simulink model "TV_LQR"  (R2024a)
settings: Solver=ode45  StartTime=0.0  StopTime=5*2.7499  MaxStep=0.001  RelTol=1e-10  AbsTol=1e-12
values from neighbouring files (symbols this model uses):
  K_all = zeros(3,6,N)    [time_varying_K_t.m]
  t_ref = data(:,1)    [compute_K.m]    (also in time_varying_K_t.m)
  t_vec = t_sol    [time_varying_K_t.m]
  vx_ref = X(:,4)    [compute_K.m]    (also in time_varying_K_t.m = X_ref(:,4))
  vy_ref = X(:,5)    [compute_K.m]    (also in time_varying_K_t.m = X_ref(:,5))
  vz_ref = X(:,6)    [compute_K.m]    (also in time_varying_K_t.m = X_ref(:,6))
  x0 = X(1,:)'    [compute_K.m]    (also in continuation.m = [r0;v0]; controlled_and_reference_orbit.m = [r0;v0]; halo_orbit_richardson.m = [r0;v0]; time_varying_K_t.m = X_ref(1,:)')
  x_ref = X(:,1)    [compute_K.m]    (also in time_varying_K_t.m = X_ref(:,1))
  y_ref = X(:,2)    [compute_K.m]    (also in time_varying_K_t.m = X_ref(:,2))
  z_ref = X(:,3)    [compute_K.m]    (also in time_varying_K_t.m = X_ref(:,3))
libraries: simulink x6
settings Model: Creator=MEGHNA  LastModifiedBy=MEGHNA
settings SolverCC: AutoScaleAbsTol=off

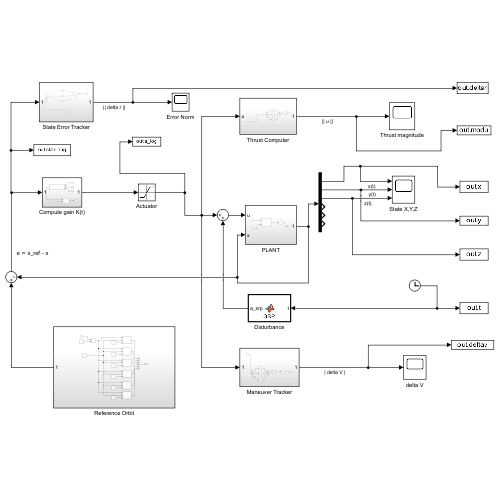
[thumbnail: Simulink's stored preview of the top-level diagram]
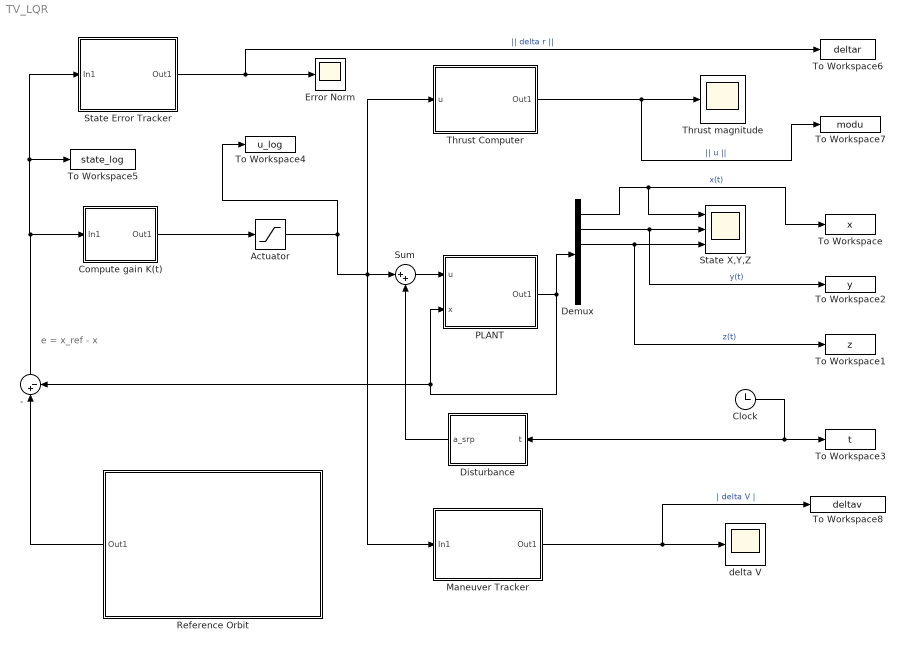
== system TV_LQR ==
  note: e = x_ref - x
  - : Sum  Inputs=|+-
  Actuator : Saturate  UpperLimit=5e-4  LowerLimit=-5e-4  LinearizeAsGain=off
  Clock : Clock
  Compute gain K(t) : Subsystem
  Demux : Demux  Outputs=6
  Disturbance : MATLAB Function  TreatAsAtomicUnit=on
  Error Norm : Scope
  Maneuver Tracker : Subsystem
  PLANT : Subsystem
  Reference Orbit : Subsystem
  State Error Tracker : Subsystem
  State X,Y,Z : Scope  NumInputPorts=3
  Sum : Sum  Inputs=|++
  Thrust Computer : Subsystem
  Thrust magnitude : Scope
  To Workspace : ToWorkspace  VariableName=x  SampleTime=-1
  To Workspace1 : ToWorkspace  VariableName=z  SampleTime=-1
  To Workspace2 : ToWorkspace  VariableName=y  SampleTime=-1
  To Workspace3 : ToWorkspace  VariableName=t  SampleTime=-1
  To Workspace4 : ToWorkspace  VariableName=u_log  SampleTime=-1
  To Workspace5 : ToWorkspace  VariableName=state_log  SampleTime=-1
  To Workspace6 : ToWorkspace  VariableName=deltar  SampleTime=-1
  To Workspace7 : ToWorkspace  VariableName=modu  SampleTime=-1
  To Workspace8 : ToWorkspace  VariableName=deltav  SampleTime=-1
  delta V : Scope
  wires:
  -/1 -> State Error Tracker/1(In1), To Workspace5/1, Compute gain K(t)/1(In1)
  Demux/1 -> To Workspace/1, State X,Y,Z/1  "x(t)"
  Demux/2 -> To Workspace2/1, State X,Y,Z/2  "y(t)"
  Demux/3 -> To Workspace1/1, State X,Y,Z/3  "z(t)"
  State Error Tracker/1(Out1) -> To Workspace6/1, Error Norm/1  "|| delta r ||"
  Maneuver Tracker/1(Out1) -> To Workspace8/1, delta V/1  "| delta V |"
  Actuator/1 -> Maneuver Tracker/1(In1), Sum/1, Thrust Computer/1(u), To Workspace4/1
  Thrust Computer/1(Out1) -> To Workspace7/1, Thrust magnitude/1  "|| u ||"
  Reference Orbit/1(Out1) -> -/1
  Clock/1 -> Disturbance/1(t), To Workspace3/1
  Sum/1 -> PLANT/1(u)
  Disturbance/1(a_srp) -> Sum/2
  PLANT/1(Out1) -> Demux/1, PLANT/2(x), -/2
  Compute gain K(t)/1(Out1) -> Actuator/1

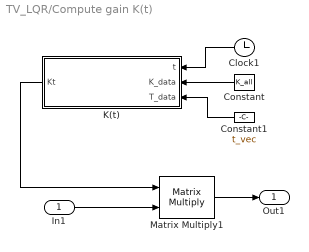
== system TV_LQR/Compute gain K(t) ==
  In1 : Inport
  Clock1 : Clock
  Constant : Constant  Value=K_all  SampleTime=-1
  Constant1 : Constant  Value=t_vec  SampleTime=-1
  K(t) : MATLAB Function  TreatAsAtomicUnit=on  SystemSampleTime=0.002
  Matrix Multiply1 : Product  Multiplication=Matrix(*)
  Out1 : Outport
  wires:
  Clock1/1 -> K(t)/1(t)
  In1/1 -> Matrix Multiply1/2
  Matrix Multiply1/1 -> Out1/1
  K(t)/1(Kt) -> Matrix Multiply1/1
  Constant/1 -> K(t)/2(K_data)
  Constant1/1 -> K(t)/3(T_data)

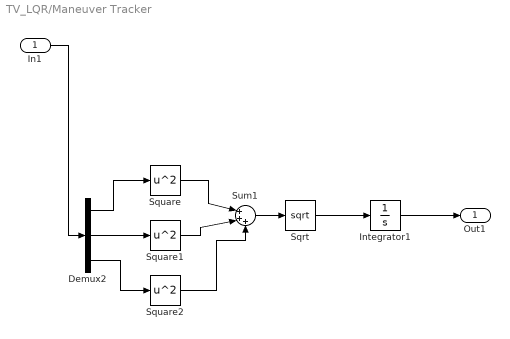
== system TV_LQR/Maneuver Tracker ==
  In1 : Inport
  Demux2 : Demux  Outputs=3
  Integrator1 : Integrator
  Sqrt : Sqrt
  Square : Math  Operator=square
  Square1 : Math  Operator=square
  Square2 : Math  Operator=square
  Sum1 : Sum  Inputs=|+++
  Out1 : Outport
  wires:
  Demux2/2 -> Square1/1
  Demux2/1 -> Square/1
  Square2/1 -> Sum1/3
  Square1/1 -> Sum1/2
  Sum1/1 -> Sqrt/1
  Square/1 -> Sum1/1
  Demux2/3 -> Square2/1
  Sqrt/1 -> Integrator1/1
  In1/1 -> Demux2/1
  Integrator1/1 -> Out1/1

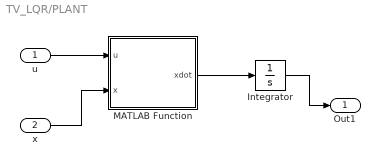
== system TV_LQR/PLANT ==
  u : Inport
  x : Inport  Port=2
  Integrator : Integrator  InitialCondition=x0
  MATLAB Function : MATLAB Function  TreatAsAtomicUnit=on
  Out1 : Outport
  wires:
  MATLAB Function/1(xdot) -> Integrator/1
  x/1 -> MATLAB Function/2(x)
  Integrator/1 -> Out1/1
  u/1 -> MATLAB Function/1(u)

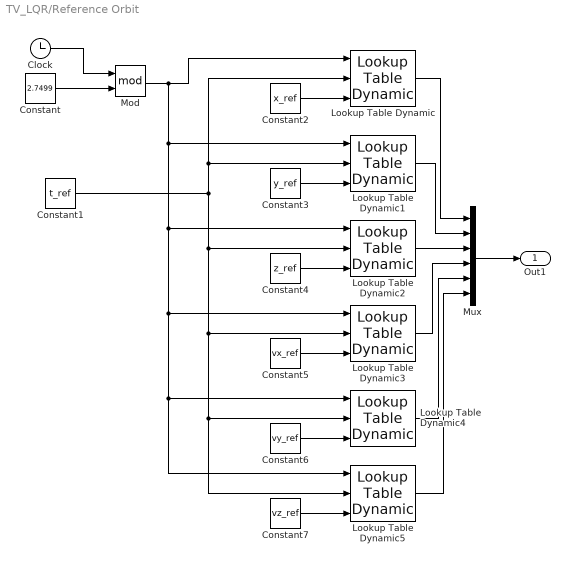
== system TV_LQR/Reference Orbit ==
  Clock : Clock
  Constant : Constant  Value=2.7499
  Constant1 : Constant  Value=t_ref
  Constant2 : Constant  Value=x_ref
  Constant3 : Constant  Value=y_ref
  Constant4 : Constant  Value=z_ref
  Constant5 : Constant  Value=vx_ref
  Constant6 : Constant  Value=vy_ref
  Constant7 : Constant  Value=vz_ref
  Lookup Table Dynamic{,1..5} (6 alike) : simulink/Lookup Tables/Lookup Table Dynamic  LookUpMeth=Interpolation-Use End Values  OutDataType=fixdt('double')  OutScaling=[]  OutputDataTypeScalingMode=Specify via dialog  OutDataTypeStr=double  DoSatur=off
  Mod : Math  Operator=mod
  Mux : Mux  Inputs=6
  Out1 : Outport
  wires:
  Lookup Table Dynamic4/1 -> Mux/5
  Constant5/1 -> Lookup Table Dynamic3/3
  Constant1/1 -> Lookup Table Dynamic5/2, Lookup Table Dynamic4/2, Lookup Table Dynamic3/2, Lookup Table Dynamic2/2, Lookup Table Dynamic1/2, Lookup Table Dynamic/2
  Lookup Table Dynamic1/1 -> Mux/2
  Mod/1 -> Lookup Table Dynamic5/1, Lookup Table Dynamic4/1, Lookup Table Dynamic3/1, Lookup Table Dynamic2/1, Lookup Table Dynamic1/1, Lookup Table Dynamic/1
  Lookup Table Dynamic/1 -> Mux/1
  Lookup Table Dynamic2/1 -> Mux/3
  Constant2/1 -> Lookup Table Dynamic/3
  Constant3/1 -> Lookup Table Dynamic1/3
  Constant4/1 -> Lookup Table Dynamic2/3
  Lookup Table Dynamic3/1 -> Mux/4
  Mux/1 -> Out1/1
  Constant6/1 -> Lookup Table Dynamic4/3
  Constant7/1 -> Lookup Table Dynamic5/3
  Lookup Table Dynamic5/1 -> Mux/6
  Clock/1 -> Mod/1
  Constant/1 -> Mod/2

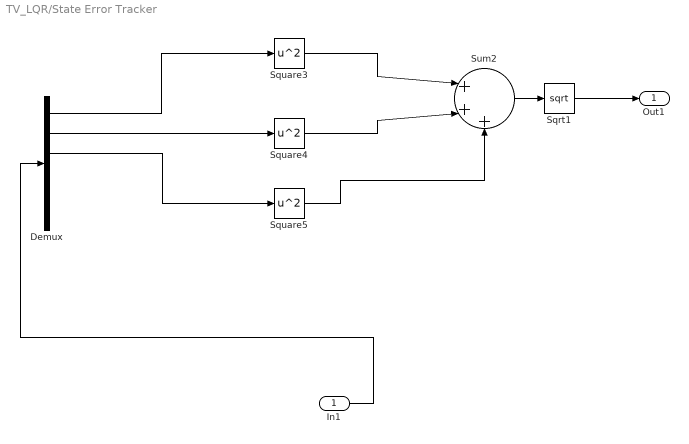
== system TV_LQR/State Error Tracker ==
  In1 : Inport
  Demux : Demux  Outputs=6
  Sqrt1 : Sqrt
  Square3 : Math  Operator=square
  Square4 : Math  Operator=square
  Square5 : Math  Operator=square
  Sum2 : Sum  Inputs=|+++
  Out1 : Outport
  wires:
  Square4/1 -> Sum2/2
  Sum2/1 -> Sqrt1/1
  Demux/2 -> Square4/1
  Demux/3 -> Square5/1
  Square3/1 -> Sum2/1
  Demux/1 -> Square3/1
  Square5/1 -> Sum2/3
  In1/1 -> Demux/1
  Sqrt1/1 -> Out1/1

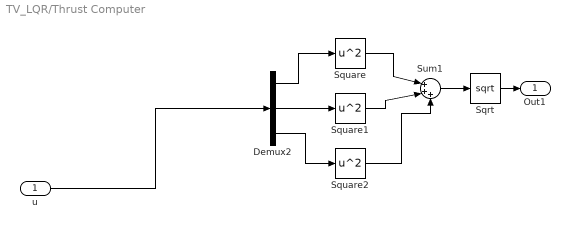
== system TV_LQR/Thrust Computer ==
  u : Inport
  Demux2 : Demux  Outputs=3
  Sqrt : Sqrt
  Square : Math  Operator=square
  Square1 : Math  Operator=square
  Square2 : Math  Operator=square
  Sum1 : Sum  Inputs=|+++
  Out1 : Outport
  wires:
  Square/1 -> Sum1/1
  u/1 -> Demux2/1
  Square2/1 -> Sum1/3
  Square1/1 -> Sum1/2
  Demux2/3 -> Square2/1
  Sum1/1 -> Sqrt/1
  Demux2/2 -> Square1/1
  Demux2/1 -> Square/1
  Sqrt/1 -> Out1/1

== matlab function TV_LQR/Compute gain K(t)/K(t) ==
  settings: updateMethod=DISCRETE  sampleTime=0.002
  data: t input size=1; Kt output size=[3 6]; K_data input size=[3 6 305]; T_data input size=[305 1]
function Kt = compute_K(t, K_data, T_data)
%#codegen

% --- FORCE FIXED OUTPUT SIZE ---
Kt = zeros(3,6);

N = 305;   % <-- HARD-CODE THIS (IMPORTANT)

T_final = T_data(N);

% periodic wrap
t = mod(t, T_final);

% --- manual index search (codegen-safe) ---
idx = 1;

for i = 1:N-1
    if t >= T_data(i) && t < T_data(i+1)
        idx = i;
        break;
    end
end

% boundary safety
if t >= T_data(N)
    idx = N-1;
end

t1 = T_data(idx);
t2 = T_data(idx+1);

K1 = K_data(:,:,idx);
K2 = K_data(:,:,idx+1);

alpha = (t - t1)/(t2 - t1);

Kt = (1-alpha)*K1 + alpha*K2;

end

== matlab function TV_LQR/PLANT/MATLAB Function ==
  data: u input double size=[3 1]; xdot output double size=[6 1]; x input double size=[6 1]
function xdot = cr3bp(u, x)

mu = 0.0121505856;

mu1 = 1-mu; % mass of larger  primary 
mu2 = mu;   % mass of smaller primary 

r1 = ((x(1)+mu2)^2 + x(2)^2 + x(3)^2)^(3/2); % r1: distance to m1   
r2 = ((x(1)-mu1)^2 + x(2)^2 + x(3)^2)^(3/2); % r2: distance to m2

xdot = zeros(6,1);

%control accelerations
ax = u(1);
ay = u(2);
az = u(3);

xdot(1) = x(4);
xdot(2) = x(5);
xdot(3) = x(6);
xdot(4) = x(1)-(mu1*(x(1)+mu2)/r1) -(mu2*(x(1)-mu1)/r2) + 2*x(5) + ax;
xdot(5) = x(2)-(mu1* x(2)/r1) -(mu2*x(2)/r2) - 2*x(4) + ay;
xdot(6) =     -(mu1* x(3)/r1) - (mu2*x(3)/r2) + az;

%tol = 1e-12;
%r1 = max(r1, tol);
%r2 = max(r2, tol);

end

== matlab function TV_LQR/Disturbance ==
  data: a_srp output; t input
function a_srp = SRP(t)

a0 = 3e-5;     % nondimensional SRP magnitude
omega = 1;      % rotation rate in CR3BP frame

sx =  cos(omega*t);
sy = -sin(omega*t);
sz =  0;

a_srp = a0 * [sx; sy; sz];

end
